simulink model "SinglePulseModel_n_20"  (R2014b)
settings: Solver=FixedStepDiscrete  StartTime=0.0  StopTime=200  RelTol=1e-3
InitFcn:
  | initialization_n_20;
StopFcn:
  | OutputPlotting;
values from neighbouring files (symbols this model uses):
  delays = tim(T,n,1:n)    [initialization.m]    (also in initialization_new.m = [10e-9, 14.33e-9, 18.66e-9]; runPulsePickingModel.m = []; runSinglePulseModel_n_6.m; runSinglePulseModel_n_8.m)
libraries: BlockLib x63, dspsrcs4 x1
settings Model: Creator=kunalmenda  LastModifiedBy=kunalmenda

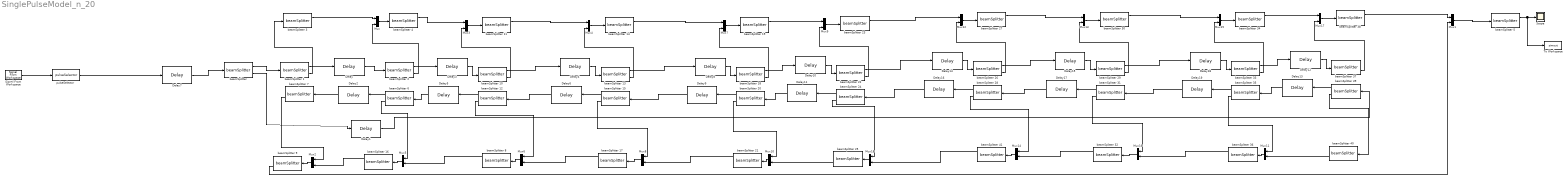
== system SinglePulseModel_n_20 ==
  Delay : BlockLib/Delay  DelayAmt=delays(2)-delays(1)
  Delay1 : BlockLib/Delay  DelayAmt=delays(11)-delays(1)
  Delay10 : BlockLib/Delay  DelayAmt=delays(6)-delays(5)
  Delay11 : BlockLib/Delay  DelayAmt=delays(6)-delays(5)
  Delay12 : BlockLib/Delay  DelayAmt=delays(10)-delays(9)
  Delay13 : BlockLib/Delay  DelayAmt=delays(10)-delays(9)
  Delay14 : BlockLib/Delay  DelayAmt=delays(7)-delays(6)
  Delay15 : BlockLib/Delay  DelayAmt=delays(8)-delays(7)
  Delay16 : BlockLib/Delay  DelayAmt=delays(7)-delays(6)
  Delay17 : BlockLib/Delay  DelayAmt=delays(8)-delays(7)
  Delay18 : BlockLib/Delay  DelayAmt=delays(9)-delays(8)
  Delay19 : BlockLib/Delay  DelayAmt=delays(9)-delays(8)
  Delay2 : BlockLib/Delay  DelayAmt=delays(2)-delays(1)
  Delay3 : BlockLib/Delay  DelayAmt=delays(3)-delays(2)
  Delay4 : BlockLib/Delay  DelayAmt=delays(4)-delays(3)
  Delay5 : BlockLib/Delay  DelayAmt=delays(3)-delays(2)
  Delay6 : BlockLib/Delay  DelayAmt=delays(4)-delays(3)
  Delay7 : BlockLib/Delay  DelayAmt=delays(1)
  Delay8 : BlockLib/Delay  DelayAmt=delays(5)-delays(4)
  Delay9 : BlockLib/Delay  DelayAmt=delays(5)-delays(4)
  Mux{,1..18} (19 alike) : Mux  Inputs=2
  Scope : Scope
  Signal From Workspace : dspsrcs4/Signal From Workspace  X=inputsignal  Ts=1  nsamps=1  OutputAfterFinalValue=Setting to zero  ignoreOrWarnInputAndFrameLengths=off
  To Workspace : ToWorkspace  VariableName=simout  SaveFormat=Timeseries  SampleTime=-1
  beamSplitter {,1..41} (42 alike) : BlockLib/beamSplitter 
  pulseSelector : BlockLib/pulseSelector  OutputDimensions=1  PCID=1
  wires:
  "beamSplitter "/1 -> beamSplitter 1/1
  beamSplitter 2/2 -> Mux/2
  beamSplitter 3/1 -> Mux/1
  Mux/1 -> beamSplitter 4/1
  Mux1/1 -> beamSplitter 5/1
  Delay/1 -> beamSplitter 2/1
  beamSplitter 1/2 -> beamSplitter 3/1
  Delay2/1 -> beamSplitter 7/1
  beamSplitter 7/2 -> Mux2/1
  Mux2/1 -> beamSplitter 9/1
  beamSplitter 9/2 -> Mux1/2
  beamSplitter 5/1 -> To Workspace/1, Scope/1
  "beamSplitter "/2 -> Delay1/1
  beamSplitter 1/1 -> Delay/1
  beamSplitter 10/2 -> Mux3/2
  Mux3/1 -> beamSplitter 11/1
  beamSplitter 4/1 -> Mux3/1
  beamSplitter 2/1 -> Delay3/1
  Delay3/1 -> beamSplitter 10/1
  beamSplitter 12/1 -> Delay5/1
  Delay5/1 -> beamSplitter 6/1
  Mux5/1 -> beamSplitter 16/1
  beamSplitter 6/2 -> Mux5/1
  beamSplitter 8/1 -> Mux5/2
  beamSplitter 16/1 -> Mux2/2
  Delay7/1 -> "beamSplitter "/1
  beamSplitter 6/1 -> Delay2/1
  pulseSelector/1 -> Delay7/1
  Signal From Workspace/1 -> pulseSelector/1
  beamSplitter 13/2 -> Mux4/2
  Mux4/1 -> beamSplitter 14/1
  beamSplitter 11/1 -> Mux4/1
  Delay4/1 -> beamSplitter 13/1
  beamSplitter 15/1 -> Delay6/1
  Delay6/1 -> beamSplitter 12/1
  beamSplitter 12/2 -> Mux6/1
  Mux6/1 -> beamSplitter 8/1
  beamSplitter 18/2 -> Mux7/2
  Mux7/1 -> beamSplitter 19/1
  beamSplitter 14/1 -> Mux7/1
  Delay8/1 -> beamSplitter 18/1
  beamSplitter 20/1 -> Delay9/1
  Delay9/1 -> beamSplitter 15/1
  beamSplitter 10/1 -> Delay4/1
  beamSplitter 13/1 -> Delay8/1
  beamSplitter 15/2 -> Mux8/1
  Mux8/1 -> beamSplitter 17/1
  beamSplitter 22/2 -> Mux9/2
  Mux9/1 -> beamSplitter 23/1
  Delay10/1 -> beamSplitter 22/1
  beamSplitter 24/1 -> Delay11/1
  beamSplitter 19/1 -> Mux9/1
  beamSplitter 18/1 -> Delay10/1
  Delay11/1 -> beamSplitter 20/1
  Mux10/1 -> beamSplitter 21/1
  beamSplitter 20/2 -> Mux10/1
  beamSplitter 25/2 -> Mux10/2
  beamSplitter 17/1 -> Mux6/2
  beamSplitter 21/1 -> Mux8/2
  beamSplitter 26/2 -> Mux12/2
  Mux12/1 -> beamSplitter 27/1
  beamSplitter 23/1 -> Mux12/1
  Delay14/1 -> beamSplitter 26/1
  beamSplitter 28/1 -> Delay16/1
  beamSplitter 41/1 -> Mux18/2
  beamSplitter 29/2 -> Mux13/2
  Mux13/1 -> beamSplitter 30/1
  beamSplitter 27/1 -> Mux13/1
  Delay15/1 -> beamSplitter 29/1
  beamSplitter 31/1 -> Delay17/1
  Delay17/1 -> beamSplitter 28/1
  beamSplitter 28/2 -> Mux14/1
  Mux14/1 -> beamSplitter 41/1
  beamSplitter 33/2 -> Mux15/2
  Mux15/1 -> beamSplitter 34/1
  beamSplitter 30/1 -> Mux15/1
  Delay18/1 -> beamSplitter 33/1
  beamSplitter 35/1 -> Delay19/1
  Delay19/1 -> beamSplitter 31/1
  beamSplitter 26/1 -> Delay15/1
  beamSplitter 29/1 -> Delay18/1
  beamSplitter 31/2 -> Mux16/1
  Mux16/1 -> beamSplitter 32/1
  beamSplitter 37/2 -> Mux17/2
  Mux17/1 -> beamSplitter 38/1
  Delay12/1 -> beamSplitter 37/1
  beamSplitter 39/1 -> Delay13/1
  beamSplitter 39/2 -> beamSplitter 40/1
  beamSplitter 34/1 -> Mux17/1
  beamSplitter 33/1 -> Delay12/1
  Delay13/1 -> beamSplitter 35/1
  Mux11/1 -> beamSplitter 36/1
  beamSplitter 35/2 -> Mux11/1
  beamSplitter 40/2 -> Mux11/2
  beamSplitter 32/1 -> Mux14/2
  beamSplitter 36/1 -> Mux16/2
  Mux18/1 -> beamSplitter 25/1
  beamSplitter 24/2 -> Mux18/1
  beamSplitter 22/1 -> Delay14/1
  Delay16/1 -> beamSplitter 24/1
  Delay1/1 -> beamSplitter 39/1
  beamSplitter 38/1 -> Mux1/1
